simulink model "SIM300kW_3paneles"  (R2022b)
settings: Solver=ode23tb  StartTime=0.0  StopTime=1  FixedStep=(5.5555555555555558E-6)/1000  RelTol=1e-7
model workspace (MAT data in the model file):
  Ir1 = 200
  Ir2 = 1000
  Ir3 = 1000
  Sig = Simulink.Signal
  Sig.DataType = 'auto'
  Sig.Dimensions = -1
  Sig.DimensionsMode = 'auto'
  Sig.Complexity = 'auto'
  Sig.SampleTime = -1
  Sig.SamplingMode = 'auto'
  T1 = 35
  initialDuty = 0.2
undefined symbols (not defined in the file or in its folder): Cin, Cout, GainDutyPenalty, GainReward, Ir4, L, MAX_DUTTY, MIN_DUTTY, N_panels, Pmax, Pmmtstc, Req, RL, Tf, Ts, Vmp
libraries: simulink x4, spsSeriesRLCBranchLib x4, spsDiodeLib x3, spsPVArrayLib x3, spsMosfetLib x2, spsCurrentMeasurementLib x1, spsPWMGeneratorDCDCLib x1, spsParallelRLCBranchLib x1, spsVoltageMeasurementLib x1, rllib x1, spspowerguiLib x1
settings Model: SimulationMode=accelerator  Creator=MathWorks  LastModifiedBy=jfgf1
settings SolverCC: ZcThreshold=100000000  MaxConsecutiveZCs=1000000  MaxConsecutiveMinStep=10  ZeroCrossControl=EnableAll  AlgebraicLoopSolver=LineSearch  SolverResetMethod=Robust  EnableFixedStepZeroCrossing=on
settings DataIOCC: LimitDataPoints=on  SaveFormat=Array  SignalLoggingSaveFormat=ModelDataLogs
settings OptimizationCC: ExpressionDepthLimit=2147483647  LifeSpan=inf
settings DebuggingCC: UnderspecifiedInitializationDetection=Classic  MergeDetectMultiDrivingBlocksExec=none  IgnoredZcDiagnostic=none  SolverPrmCheckMsg=warning  UnconnectedInputMsg=warning  UnconnectedOutputMsg=warning  UnconnectedLineMsg=warning  AllowSymbolicDim=off  StateNameClashWarn=warning  SFUnexpectedBacktrackingDiag=warning  SFNoUnconditionalDefaultTransitionDiag=warning  SFExecutionAtInitializationDiag=none  SFMachineParentedDataDiag=warning  ArithmeticOperatorsInVariantConditions=warning
settings HardwareCC: ProdBitPerPointer=32  ProdBitPerSizeT=32  ProdBitPerPtrDiffT=32  ProdLargestAtomicFloat=None  ProdIntDivRoundTo=Undefined  ProdEndianess=Unspecified  ProdWordSize=32  ProdHWDeviceType=32-bit Generic
settings ModelReferenceCC: EnableRefExpFcnMdlSchedulingChecks=on  PropagateSignalLabelsOutOfModel=off
settings SFSimCC: SimUseLocalCustomCode=off  CustomCodeUndefinedFunction=UseInterfaceOnly
settings RTWCC: RTWUseLocalCustomCode=off  DLArmComputeVersion=19.05
settings CodeAppCC: StateflowObjectComments=on
settings GRTTargetCC: TargetLangStandard=C89/C90 (ANSI)  CombineOutputUpdateFcns=off  GRTInterface=on
settings ConfigComp: CovMetricSettings=dw  CovSaveCumulativeToWorkspaceVar=on  CovSaveSingleToWorkspaceVar=on  CovExternalEMLEnable=off  CovSFcnEnable=off
settings SimscapeCC: SimscapeNormalizeSystem=off

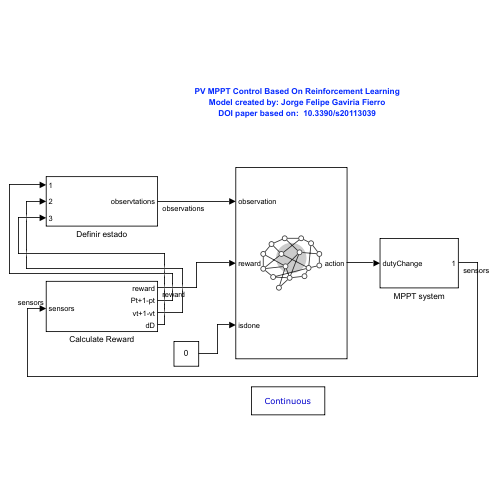
[thumbnail: Simulink's stored preview of the top-level diagram]
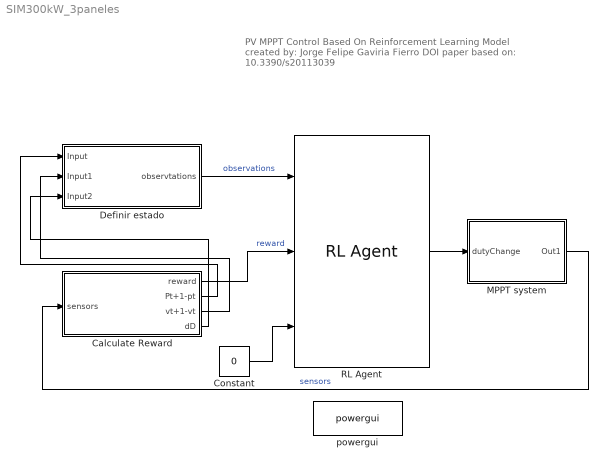
== system SIM300kW_3paneles ==
  note: PV MPPT Control Based On Reinforcement Learning
      | Model created by: Jorge Felipe Gaviria Fierro
      | DOI paper based on: 10.3390/s20113039
  Calculate Reward : Subsystem
  Constant : Constant  Value=0
  Definir estado : Subsystem
  MPPT system : Subsystem
  RL Agent : rllib/RL Agent  Agent=agentObj  ExternalActionAsInput=off  ProvideLastAction=off  ProvideCumRwd=off  TreatAsDirectFeedthrough=on  UseStrictObservationDataTypes=off
  powergui : spspowerguiLib/powergui  Priority=1  SimulationMode=Continuous  SampleTime=0.00001  frequency=60  Iterations=50  frequencyindice=0  Pbase=100e6  ErrMax=1e-4  UnitsV=kV  UnitsW=MW  buscounter=0  FunctionMessages=off  echomessages=off  EnableUseOfTLC=off  CurrentSourceSwitches=on  DisableSnubberDevices=on  DisableRonSwitches=off  DisableVfSwitches=off  DisplayEquations=off  AutomaticDiscreteSolvers=off  SolverType=Tustin/Backward Euler (TBE)  Interpol=off  ExternalGateDelay=off  methode=off  Ts=0  x0status=blocks  SPID=off  SwTol=0  HookPort=off  NonlinearTolerance=1e-4  nMaxIteration=100  ContinueOnMaxIteration=off  RestoreLinks=warning  ResistiveCurrentMeasurement=off  Frange=[0:2:500]  Ylog=off  Xlog=on  ShowGrid=off  save=off  variable=ZData  structure=0  ZoomFFT=on  StartTime=0.0  cycles=1  DisplayStyle=1  fundamental=60  FreqAxis=off  MaxFrequency=1000  frequencyindicesteady=1  RmsSteady=1  display=off
  wires:
  RL Agent/1 -> MPPT system/1(dutyChange)
  MPPT system/1(Out1) -> Calculate Reward/1(sensors)  "sensors"
  Definir estado/1(observtations) -> RL Agent/1  "observations"
  Constant/1 -> RL Agent/3
  Calculate Reward/1(reward) -> RL Agent/2  "reward"
  Calculate Reward/2(Pt+1-pt) -> Definir estado/1(Input)
  Calculate Reward/3(vt+1-vt) -> Definir estado/2(Input1)
  Calculate Reward/4(dD) -> Definir estado/3(Input2)

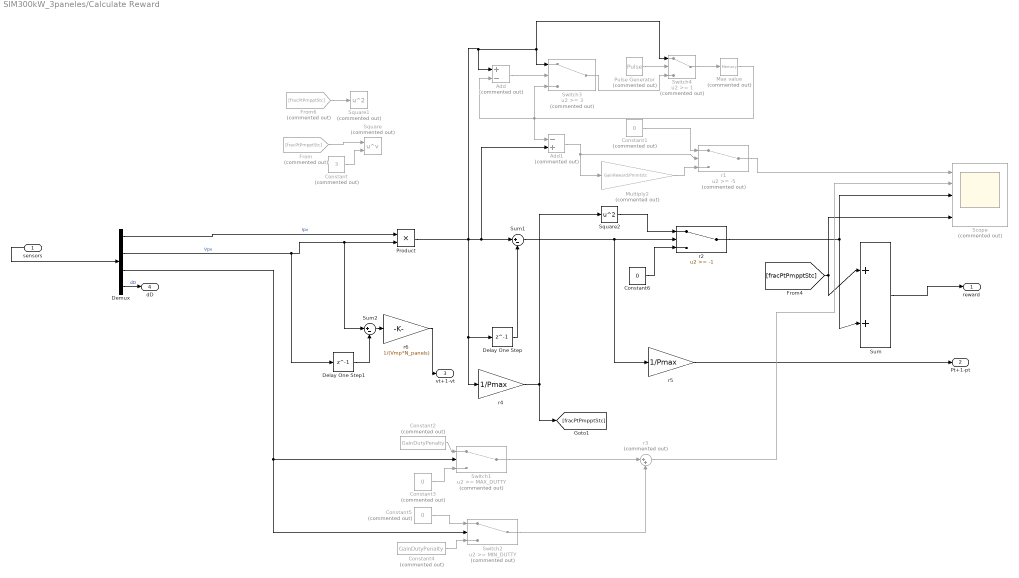
== system SIM300kW_3paneles/Calculate Reward ==
  sensors : Inport
  Add : Sum  Commented=on  Inputs=+-
  Add1 : Sum  Commented=on  Inputs=-+
  Constant : Constant  Commented=on  Value=3
  Constant1 : Constant  Commented=on  Value=0
  Constant2 : Constant  Commented=on  Value=GainDutyPenalty
  Constant3 : Constant  Commented=on  Value=0
  Constant4 : Constant  Commented=on  Value=GainDutyPenalty
  Constant5 : Constant  Commented=on  Value=0
  Constant6 : Constant  Value=0
  Delay One Step : Delay  DelayLength=1  SampleTime=Ts
  Delay One Step1 : Delay  DelayLength=1  SampleTime=Ts
  Demux : Demux
  From : From  Commented=on  GotoTag=fracPtPmpptStc
  From6 : From  Commented=on  GotoTag=fracPtPmpptStc
  Max value : Memory  Commented=on
  Multiply2 : Gain  Commented=on  Gain=GainReward/Pmmtstc
  Product : Product
  Pulse Generator : DiscretePulseGenerator  Commented=on  PulseType=Time based  Amplitude=0  Period=Tf
  Scope : Scope  Commented=on  NumInputPorts=5
  Square : Math  Commented=on  Operator=pow  OutputSignalType=real
  Square1 : Math  Commented=on  Operator=square
  Square2 : Math  Operator=square
  Sum : Sum  Inputs=|++
  Sum1 : Sum  Inputs=|+-
  Sum2 : Sum  Inputs=|+-
  Switch1 : Switch  Commented=on  Threshold=MAX_DUTTY  SaturateOnIntegerOverflow=off  InputSameDT=off
  Switch2 : Switch  Commented=on  Threshold=MIN_DUTTY  SaturateOnIntegerOverflow=off  InputSameDT=off
  Switch3 : Switch  Commented=on  Threshold=3  SaturateOnIntegerOverflow=off  InputSameDT=off
  Switch4 : Switch  Commented=on  Threshold=1  SaturateOnIntegerOverflow=off  InputSameDT=off
  r1 : Switch  Commented=on  Threshold=-5  SaturateOnIntegerOverflow=off  InputSameDT=off
  r2 : Switch  Threshold=-1  SaturateOnIntegerOverflow=off  InputSameDT=off
  r3 : Sum  Commented=on  Inputs=|++
  r4 : Gain  Gain=1/Pmax
  r5 : Gain  Gain=1/Pmax
  r6 : Gain  Gain=1/(Vmp*N_panels)
  reward : Outport
  Pt+1-pt : Outport  Port=2
  vt+1-vt : Outport  Port=3
  dD : Outport  Port=4
  wires:
  sensors/1 -> Demux/1
  Demux/1 -> Product/1  "Ipv"
  Demux/2 -> Delay One Step1/1, Sum2/1, Product/2  "Vpv"
  Sum/1 -> reward/1
  Delay One Step/1 -> Sum1/2
  Constant2/1 -> Switch1/1
  Constant3/1 -> Switch1/3
  Switch1/1 -> r3/1
  Switch2/1 -> r3/2
  Demux/3 -> Switch2/2, Switch1/2
  Max value/1 -> Add1/1, Switch3/3, Add/2
  Pulse Generator/1 -> Switch4/2
  Product/1 -> r4/1, Delay One Step/1, Sum1/1, Add1/2, Switch3/1, Switch4/1, Add/1
  Switch4/1 -> Max value/1
  Add/1 -> Switch3/2
  Add1/1 -> Multiply2/1, r1/2
  Constant1/1 -> r1/1
  Switch3/1 -> Switch4/3
  r4/1 -> Square2/1, [fracPtPmpptStc]
  From/1 -> Square/1
  [fracPtPmpptStc] -> Scope/5, Sum/1
  From6/1 -> Square1/1
  Multiply2/1 -> r1/3
  r5/1 -> Pt+1-pt/1
  Constant5/1 -> Switch2/1
  Constant4/1 -> Switch2/3
  Demux/4 -> dD/1  "dD"
  Delay One Step1/1 -> Sum2/2
  r6/1 -> vt+1-vt/1
  Sum2/1 -> r6/1
  r2/1 -> Sum/2, Scope/3
  Constant/1 -> Square/2
  Sum1/1 -> r5/1, r2/2
  Square2/1 -> r2/1
  r3/1 -> Scope/2
  Constant6/1 -> r2/3
  r1/1 -> Scope/1

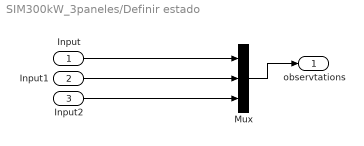
== system SIM300kW_3paneles/Definir estado ==
  Input : Inport
  Input1 : Inport  Port=2
  Input2 : Inport  Port=3
  Mux : Mux  Inputs=3
  observtations : Outport
  wires:
  Mux/1 -> observtations/1
  Input1/1 -> Mux/2
  Input/1 -> Mux/1
  Input2/1 -> Mux/3

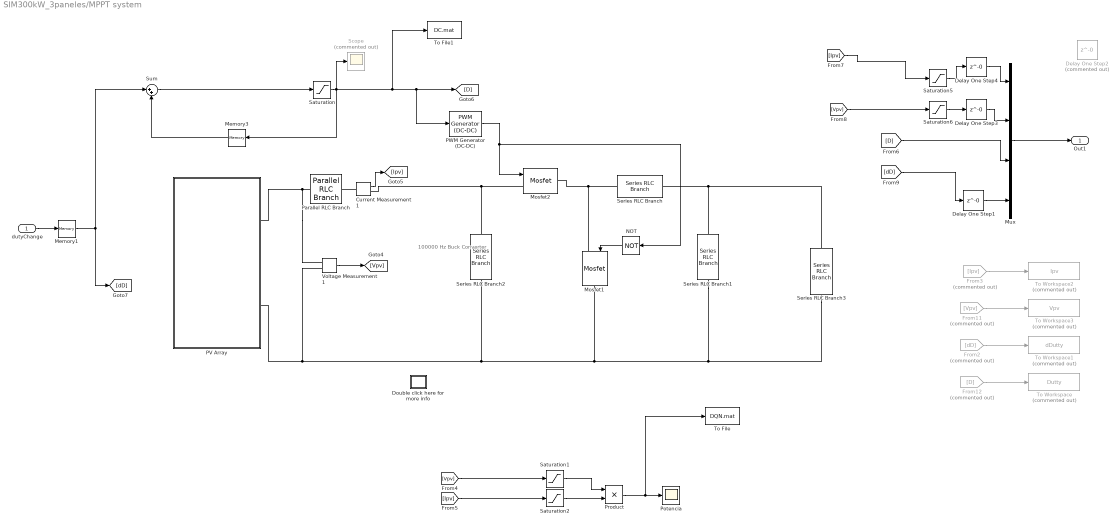
== system SIM300kW_3paneles/MPPT system ==
  note: 100000 Hz
      | Buck Converter
  dutyChange : Inport
  Current Measurement1 : spsCurrentMeasurementLib/Current Measurement  PhasorSimulation=off  OutputType=Complex  PSBequivalent=0
  Delay One Step1 : Delay  DelayLength=0  SampleTime=Ts
  Delay One Step2 : Delay  Commented=on  DelayLength=0  SampleTime=Ts
  Delay One Step3 : Delay  DelayLength=0  SampleTime=Ts
  Delay One Step4 : Delay  DelayLength=0  SampleTime=Ts
  Double click here for more info : Subsystem
      settings: OpenFcn=showdemo(bdroot(gcb))
      mask Display: disp('?')
  From11 : From  Commented=on  GotoTag=Vpv
  From12 : From  Commented=on  GotoTag=D
  From2 : From  Commented=on  GotoTag=dD
  From3 : From  Commented=on  GotoTag=Ipv
  Memory1 : Memory  InheritSampleTime=on
  Memory3 : Memory  InitialCondition=initialDuty  InheritSampleTime=on
  Mosfet1 : spsMosfetLib/Mosfet  Ron=Ron  Lon=0  Rd=0.01  Vfd=0  IC=0  Rs=1e5  Cs=inf  Measurements=off
  Mosfet2 : spsMosfetLib/Mosfet  Ron=Ron  Lon=0  Rd=0.01  Vfd=0  IC=0  Rs=1e5  Cs=inf  Measurements=off
  Mux : Mux
  NOT : Logic  Operator=NOT  IconShape=distinctive  AllPortsSameDT=off  OutDataTypeStr=boolean
  PV Array : Subsystem
  PWM Generator (DC-DC) : spsPWMGeneratorDCDCLib/PWM Generator (DC-DC)  Fsw=fs  Ts=0
  Parallel RLC Branch : spsParallelRLCBranchLib/Parallel RLC Branch  LConnTagsString=a  RConnTagsString=__new0  BranchType=R  Resistance=0.16  Inductance=1e-3  SetiL0=off  InitialCurrent=0  Capacitance=1e-6  Setx0=off  InitialVoltage=0  Measurements=None
  Potencia : Scope
  Product : Product
  Saturation : Saturate  UpperLimit=MAX_DUTTY  LowerLimit=MIN_DUTTY
  Saturation1 : Saturate  UpperLimit=1000000000000  LowerLimit=0
  Saturation2 : Saturate  UpperLimit=1000000000000  LowerLimit=0
  Saturation5 : Saturate  UpperLimit=1000000000000  LowerLimit=0
  Saturation6 : Saturate  UpperLimit=10000000000000000  LowerLimit=0
  Scope : Scope  Commented=on
  Series RLC Branch : spsSeriesRLCBranchLib/Series RLC Branch  LConnTagsString=__new0  RConnTagsString=__new0  BranchType=RL  Resistance=RL  Inductance=L  SetiL0=off  InitialCurrent=0  Capacitance=1e-6  Setx0=off  InitialVoltage=0  Measurements=None
  Series RLC Branch1 : spsSeriesRLCBranchLib/Series RLC Branch  LConnTagsString=__new0  RConnTagsString=__new0  BranchType=C  Resistance=0.001  Inductance=1e-3  SetiL0=off  InitialCurrent=0  Capacitance=Cout  Setx0=off  InitialVoltage=0  Measurements=None
  Series RLC Branch2 : spsSeriesRLCBranchLib/Series RLC Branch  LConnTagsString=__new0  RConnTagsString=__new0  BranchType=C  Resistance=0.005  Inductance=1e-3  SetiL0=off  InitialCurrent=0  Capacitance=Cin  Setx0=off  InitialVoltage=0  Measurements=None
  Series RLC Branch3 : spsSeriesRLCBranchLib/Series RLC Branch  LConnTagsString=__new0  RConnTagsString=__new0  BranchType=R  Resistance=Req  Inductance=1e-3  SetiL0=off  InitialCurrent=0  Capacitance=1e-6  Setx0=off  InitialVoltage=0  Measurements=None
  Sum : Sum  Inputs=|++
  To File : ToFile  Filename=DQN.mat  SaveFormat=Timeseries
  To File1 : ToFile  Filename=DC.mat  SaveFormat=Timeseries  SampleTime=Ts
  To Workspace : ToWorkspace  Commented=on  VariableName=Dutty  SampleTime=0.01
      settings: Save2DSignal=2-D array (concatenate along first dimension)
  To Workspace1 : ToWorkspace  Commented=on  VariableName=dDutty  SampleTime=0.01
      settings: Save2DSignal=2-D array (concatenate along first dimension)
  To Workspace2 : ToWorkspace  Commented=on  VariableName=Ipv  SampleTime=0.01
      settings: Save2DSignal=2-D array (concatenate along first dimension)
  To Workspace3 : ToWorkspace  Commented=on  VariableName=Vpv  SampleTime=0.01
      settings: Save2DSignal=2-D array (concatenate along first dimension)
  Voltage Measurement1 : spsVoltageMeasurementLib/Voltage Measurement  PhasorSimulation=off  OutputType=Complex  PSBequivalent=0
  Out1 : Outport
  wires:
  dutyChange/1 -> Memory1/1
  Current Measurement1/1 -> [Ipv]
  Voltage Measurement1/1 -> [Vpv]
  Mux/1 -> Out1/1
  [dD] -> Delay One Step1/1
  Memory1/1 -> Sum/1, [dD]
  Memory3/1 -> Sum/2
  [Vpv] -> Saturation1/1
  [Ipv] -> Saturation2/1
  Sum/1 -> Saturation/1
  Product/1 -> To File/1, Potencia/1
  Saturation/1 -> Scope/1, To File1/1, PWM Generator (DC-DC)/1, [D], Memory3/1
  PWM Generator (DC-DC)/1 -> Mosfet2/1, NOT/1
  NOT/1 -> Mosfet1/1
  From2/1 -> To Workspace1/1
  From11/1 -> To Workspace3/1
  From3/1 -> To Workspace2/1
  From12/1 -> To Workspace/1
  Saturation1/1 -> Product/1
  Saturation2/1 -> Product/2
  [Ipv] -> Saturation5/1
  [Vpv] -> Saturation6/1
  Saturation6/1 -> Delay One Step3/1
  Delay One Step1/1 -> Mux/4
  [D] -> Mux/3
  Delay One Step3/1 -> Mux/2
  Delay One Step4/1 -> Mux/1
  Saturation5/1 -> Delay One Step4/1
  connections:
  Series RLC Branch1/RConn1 -- Series RLC Branch3/RConn1 -- PV Array/RConn2 -- Voltage Measurement1/LConn2 -- Series RLC Branch2/RConn1 -- Mosfet1/RConn1
  Series RLC Branch1/LConn1 -- Series RLC Branch3/LConn1 -- Series RLC Branch/RConn1
  Series RLC Branch/LConn1 -- Mosfet2/RConn1 -- Mosfet1/LConn1
  Series RLC Branch2/LConn1 -- Mosfet2/LConn1 -- Current Measurement1/RConn1
  PV Array/RConn1 -- Parallel RLC Branch/LConn1 -- Voltage Measurement1/LConn1
  Current Measurement1/LConn1 -- Parallel RLC Branch/RConn1

== system SIM300kW_3paneles/MPPT system/Double click here for more info ==

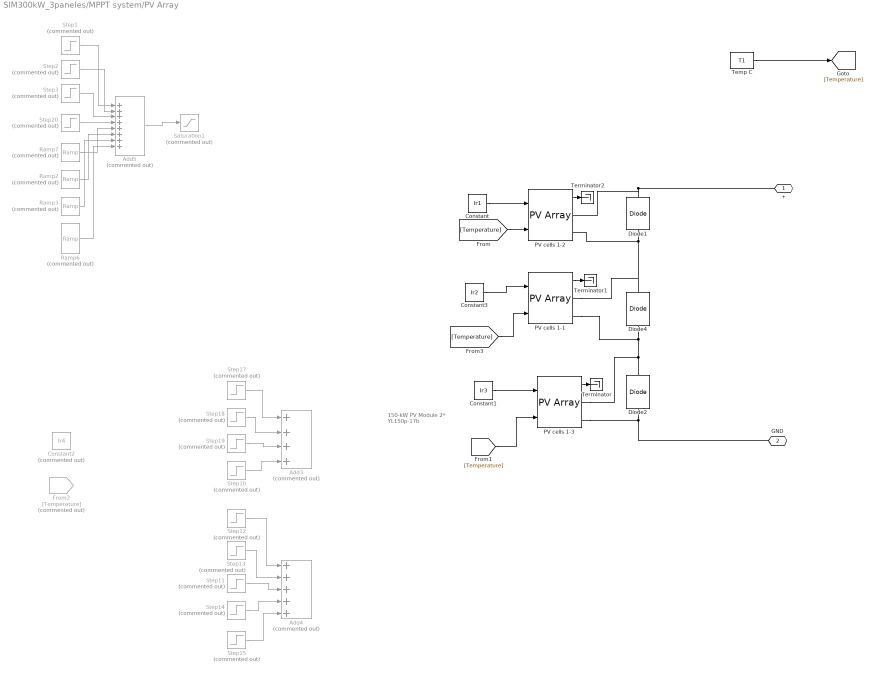
== system SIM300kW_3paneles/MPPT system/PV Array ==
  note: 150-kW  PV Module
      | 2* YL150p-17b
  Add3 : Sum  Commented=on  Inputs=++++
  Add4 : Sum  Commented=on  Inputs=+++++
  Add5 : Sum  Commented=on  Inputs=++++++++
  Constant : Constant  Value=Ir1
  Constant1 : Constant  Value=Ir3
  Constant2 : Constant  Commented=on  Value=Ir4
  Constant3 : Constant  Value=Ir2
  Diode1 : spsDiodeLib/Diode  Ron=0.001  Lon=0  Vf=0.5  IC=0  UseSnubber=off  Rs=1e5*inf  Cs=inf  Measurements=off
  Diode2 : spsDiodeLib/Diode  Ron=0.001  Lon=0  Vf=0.5  IC=0  UseSnubber=off  Rs=1e5*inf  Cs=inf  Measurements=off
  Diode4 : spsDiodeLib/Diode  Ron=0.001  Lon=0  Vf=0.5  IC=0  UseSnubber=off  Rs=1e5*inf  Cs=inf  Measurements=off
  From2 : From  Commented=on  GotoTag=Temperature
  PV cells 1-1 : spsPVArrayLib/PV Array  Npar=1  Nser=1  PlotType=array @ 1000 W/m2 & specified temperatures  S_vec="[ 1000  500  100 ]"  Temp_C_vec=[ 20 ]  ModuleName=User-defined  PlotWhenSelected=off  Pm=83.83  Ncell=20  Voc=37.3/3  Isc=8.6  Vm=30.3/3  Im=8.3  beta_Voc_pc=-0.129  alpha_Isc_pc=0.044  beta_Voc=-0.016039  alpha_Isc=0.003784  IL=8.6716  I0=1.726e-15  nI=0.66942  Rsh=199.8499  Rs=0.14456  RobustModel=off  RobustCellTemperature=25  BAL=on  Tc=1e-5  Tfilter=5e-5
  PV cells 1-2 : spsPVArrayLib/PV Array  Npar=1  Nser=1  PlotType=array @ 1000 W/m2 & specified temperatures  S_vec="[ 1000  500  100 ]"  Temp_C_vec=[ 20 ]  ModuleName=User-defined  PlotWhenSelected=off  Pm=83.83  Ncell=20  Voc=37.3/3  Isc=8.6  Vm=30.3/3  Im=8.3  beta_Voc_pc=-0.129  alpha_Isc_pc=0.044  beta_Voc=-0.016039  alpha_Isc=0.003784  IL=8.6716  I0=1.726e-15  nI=0.66942  Rsh=199.8499  Rs=0.14456  RobustModel=off  RobustCellTemperature=25  BAL=on  Tc=1e-5  Tfilter=5e-5
  PV cells 1-3 : spsPVArrayLib/PV Array  Npar=1  Nser=1  PlotType=array @ 1000 W/m2 & specified temperatures  S_vec="[ 1000  500  100 ]"  Temp_C_vec=[ 20 ]  ModuleName=User-defined  PlotWhenSelected=off  Pm=83.83  Ncell=20  Voc=37.3/3  Isc=8.6  Vm=30.3/3  Im=8.3  beta_Voc_pc=-0.129  alpha_Isc_pc=0.044  beta_Voc=-0.016039  alpha_Isc=0.003784  IL=8.6716  I0=1.726e-15  nI=0.66942  Rsh=199.8499  Rs=0.14456  RobustModel=off  RobustCellTemperature=25  BAL=on  Tc=1e-5  Tfilter=5e-5
  Ramp2 : simulink/Sources/Ramp  Commented=on  slope=-100  start=5  InitialOutput=0
  Ramp3 : simulink/Sources/Ramp  Commented=on  slope=-100  start=6  InitialOutput=0
  Ramp6 : simulink/Sources/Ramp  Commented=on  slope=100  start=7  InitialOutput=0
  Ramp7 : simulink/Sources/Ramp  Commented=on  slope=100  start=2.5  InitialOutput=0
  Saturation1 : Saturate  Commented=on  UpperLimit=1000  LowerLimit=0
  Step1 : Step  Commented=on  Time=0  After=1000  SampleTime=0
  Step10 : Step  Commented=on  Time=2  After=250  SampleTime=0
  Step11 : Step  Commented=on  Time=2  After=100  SampleTime=0
  Step12 : Step  Commented=on  Time=0  After=1000  SampleTime=0
  Step13 : Step  Commented=on  Time=0.5  After=-800  SampleTime=0
  Step14 : Step  Commented=on  Time=1.5  After=-100  SampleTime=0
  Step15 : Step  Commented=on  Time=1.5  After=200  SampleTime=0
  Step17 : Step  Commented=on  Time=0  After=1000  SampleTime=0
  Step18 : Step  Commented=on  After=-700  SampleTime=0
  Step19 : Step  Commented=on  Time=1.5  After=-400  SampleTime=0
  Step2 : Step  Commented=on  After=-100  SampleTime=0
  Step20 : Step  Commented=on  Time=2  After=-300  SampleTime=0
  Step3 : Step  Commented=on  Time=1.5  After=-100  SampleTime=0
  Temp C : Constant  Value=T1
  Terminator : Terminator
  Terminator1 : Terminator
  Terminator2 : Terminator
  + : PMIOPort  Side=Right
  GND : PMIOPort  Port=2  Side=Right
  wires:
  Temp C/1 -> [Temperature]
  [Temperature] -> PV cells 1-2/2
  Step11/1 -> Add4/3
  Step14/1 -> Add4/4
  Step17/1 -> Add3/1
  Step18/1 -> Add3/2
  Step10/1 -> Add3/4
  Step19/1 -> Add3/3
  Step13/1 -> Add4/2
  Step12/1 -> Add4/1
  Step15/1 -> Add4/5
  [Temperature] -> PV cells 1-1/2
  PV cells 1-3/1 -> Terminator/1
  PV cells 1-1/1 -> Terminator1/1
  PV cells 1-2/1 -> Terminator2/1
  Ramp3/1 -> Add5/7
  Step3/1 -> Add5/3
  Step1/1 -> Add5/1
  Ramp6/1 -> Add5/8
  Step20/1 -> Add5/4
  Step2/1 -> Add5/2
  Ramp7/1 -> Add5/5
  Add5/1 -> Saturation1/1
  Ramp2/1 -> Add5/6
  [Temperature] -> PV cells 1-3/2
  Constant/1 -> PV cells 1-2/1
  Constant3/1 -> PV cells 1-1/1
  Constant1/1 -> PV cells 1-3/1
  connections:
  PV cells 1-1/RConn1 -- Diode4/RConn1 -- Diode1/LConn1 -- PV cells 1-2/RConn2
  +/RConn1 -- PV cells 1-2/RConn1 -- Diode1/RConn1
  GND/RConn1 -- PV cells 1-3/RConn2 -- Diode2/LConn1
  Diode4/LConn1 -- PV cells 1-1/RConn2 -- PV cells 1-3/RConn1 -- Diode2/RConn1
